simulink model "GalvoModel_thesis"  (R2015a)
settings: Solver=ode45  StartTime=0.0  StopTime=10.0  RelTol=1e-3
settings Model: Creator=mainster  LastModifiedBy=mainster
settings OptimizationCC: InlineParams=on  BufferReuse=off
settings DebuggingCC: UnderspecifiedInitializationDetection=Classic  MergeDetectMultiDrivingBlocksExec=none  SolverPrmCheckMsg=warning  StateNameClashWarn=warning  InitInArrayFormatMsg=none

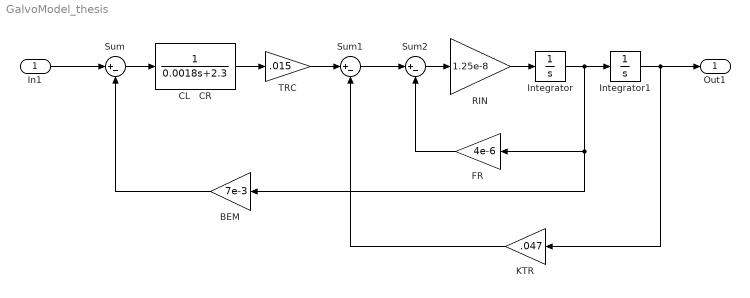
== system GalvoModel_thesis ==
  In1 : Inport
  BEM : Gain  Gain=7e-3
  CL   CR : TransferFcn  Denominator=[0.0018 2.3]
  FR : Gain  Gain=4e-6
  Integrator : Integrator
  Integrator1 : Integrator
  KTR : Gain  Gain=.047
  RIN : Gain  Gain=1.25e-8
  Sum : Sum  Inputs=|+-
  Sum1 : Sum  Inputs=|+-
  Sum2 : Sum  Inputs=|+-
  TRC : Gain  Gain=.015
  Out1 : Outport
  wires:
  In1/1 -> Sum/1
  Sum/1 -> CL   CR/1
  CL   CR/1 -> TRC/1
  TRC/1 -> Sum1/1
  Sum1/1 -> Sum2/1
  Sum2/1 -> RIN/1
  RIN/1 -> Integrator/1
  Integrator/1 -> BEM/1, FR/1, Integrator1/1
  Integrator1/1 -> KTR/1, Out1/1
  FR/1 -> Sum2/2
  BEM/1 -> Sum/2
  KTR/1 -> Sum1/2
